simulink model "Truck_model_step"  (R2025a)
settings: Solver=VariableStepAuto  StartTime=0.0  StopTime=30  RelTol=1e-3
values from neighbouring files (symbols this model uses):
  A = [zeros(10) eye(10) ... (first row only)    [New_method_with_static_Equilibrium.m]    (also in PeakForce_and_Amp.m; Rough_work.m = [0 1 0 0 0 0 0 0 0 0 0 0 0 0 0 0 0 0 0 0; Rough_work_sweep.m = [0 1 0 0 0 0 0 0 0 0 0 0 0 0 0 0 0 0 0 0)
  B = [0 0 0 0 ... (first row only)    [New_method_with_static_Equilibrium.m]    (also in PeakForce_and_Amp.m; Rough_work.m; Rough_work_sweep.m)
  C = [-(Csf+Csr+Csd) Csf Csr (-Csr*lr+Csf*lf-Csd*a1) 0 0 0 0 Csd -Csd*lfd ... (first row only)    [New_method_with_static_Equilibrium.m]    (also in PeakForce_and_Amp.m; Rough_work.m = eye(20); Rough_work_sweep.m = eye(20))
  D = zeros(20,4)    [New_method_with_static_Equilibrium.m]    (also in PeakForce_and_Amp.m; Rough_work.m; Rough_work_sweep.m)
  t1 = s1/Vx    (= 0.06825)    [New_method_with_static_Equilibrium.m]    (also in PeakForce_and_Amp.m = s1/Vx; Rough_work.m = 0.1365; Rough_work_sweep.m = s1/Vx)
  t2 = s2/Vx    (= 0.34175)    [New_method_with_static_Equilibrium.m]    (also in PeakForce_and_Amp.m = s2/Vx; Rough_work.m = 0.6835; Rough_work_sweep.m = s2/Vx)
  t3 = s3/Vx    (= 0.66575)    [New_method_with_static_Equilibrium.m]    (also in PeakForce_and_Amp.m = s3/Vx; Rough_work.m = 1.3315; Rough_work_sweep.m = s3/Vx)
  t4 = s4/Vx    (= 1.01325)    [New_method_with_static_Equilibrium.m]    (also in PeakForce_and_Amp.m = s4/Vx; Rough_work.m = 2.0265; Rough_work_sweep.m = s4/Vx)
settings Model: Creator=lenovo  LastModifiedBy=lenovo

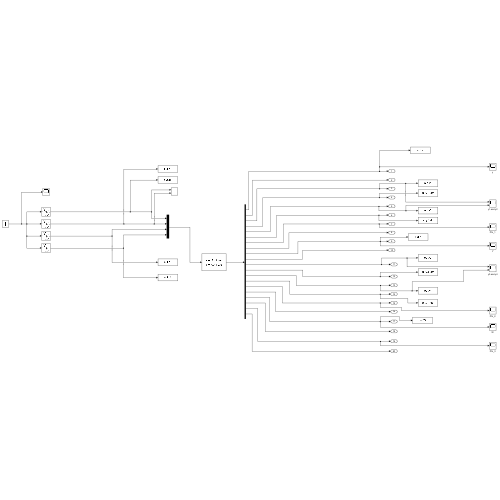
[thumbnail: Simulink's stored preview of the top-level diagram]
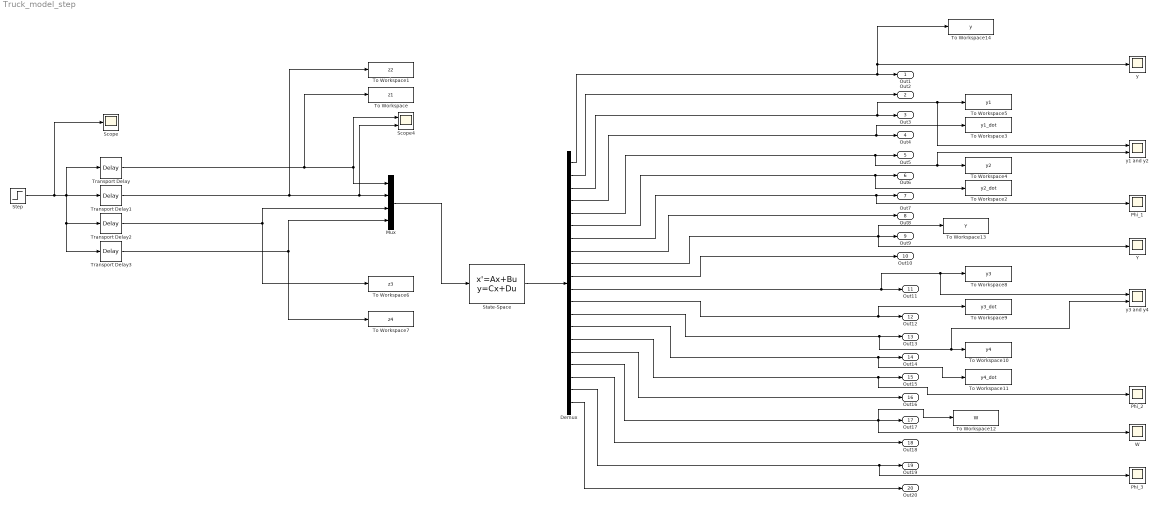
== system Truck_model_step ==
  Demux : Demux  Outputs=20
  Mux : Mux
  Phi_1 : Scope
      settings: ActiveDisplayYMinimum=-0.25192544075249879  ActiveDisplayYMaximum=0.21768735206441114  DataLoggingVariableName=ScopeData2
  Phi_2 : Scope
      settings: ActiveDisplayYMinimum=-0.0014235134101191549  ActiveDisplayYMaximum=0.0014402375247128129  DataLoggingVariableName=ScopeData9
  Phi_3 : Scope
      settings: ActiveDisplayYMinimum=-0.1066435087188474  ActiveDisplayYMaximum=0.11421754881493598  DataLoggingVariableName=ScopeData7
  Scope : Scope
      settings: ActiveDisplayYMinimum=-0.0020586486151432937  ActiveDisplayYMaximum=0.10161430322660607  DataLoggingVariableName=ScopeData8
  Scope4 : Scope  NumInputPorts=2
      settings: ActiveDisplayYMinimum=-1  ActiveDisplayYMaximum=1  DataLoggingVariableName=ScopeData4
  State-Space : StateSpace  A=A  B=B  C=C  D=D  InitialCondition=0
  Step : Step  After=0.03  SampleTime=0
  To Workspace : ToWorkspace  VariableName=z1  SaveFormat=Timeseries  SampleTime=-1
  To Workspace1 : ToWorkspace  VariableName=z2  SaveFormat=Timeseries  SampleTime=-1
  To Workspace10 : ToWorkspace  VariableName=y4  SaveFormat=Timeseries  SampleTime=-1
  To Workspace11 : ToWorkspace  VariableName=y4_dot  SaveFormat=Timeseries  SampleTime=-1
  To Workspace12 : ToWorkspace  VariableName=W  SaveFormat=Timeseries  SampleTime=-1
  To Workspace13 : ToWorkspace  VariableName=Y  SaveFormat=Timeseries  SampleTime=-1
  To Workspace14 : ToWorkspace  VariableName=y  SaveFormat=Timeseries  SampleTime=-1
  To Workspace2 : ToWorkspace  VariableName=y2_dot  SaveFormat=Timeseries  SampleTime=-1
  To Workspace3 : ToWorkspace  VariableName=y1_dot  SaveFormat=Timeseries  SampleTime=-1
  To Workspace4 : ToWorkspace  VariableName=y2  SaveFormat=Timeseries  SampleTime=-1
  To Workspace5 : ToWorkspace  VariableName=y1  SaveFormat=Timeseries  SampleTime=-1
  To Workspace6 : ToWorkspace  VariableName=z3  SaveFormat=Timeseries  SampleTime=-1
  To Workspace7 : ToWorkspace  VariableName=z4  SaveFormat=Timeseries  SampleTime=-1
  To Workspace8 : ToWorkspace  VariableName=y3  SaveFormat=Timeseries  SampleTime=-1
  To Workspace9 : ToWorkspace  VariableName=y3_dot  SaveFormat=Timeseries  SampleTime=-1
  Transport Delay : TransportDelay  DelayTime=t1  BufferSize=102400
  Transport Delay1 : TransportDelay  DelayTime=t2  BufferSize=102400
  Transport Delay2 : TransportDelay  DelayTime=t3  BufferSize=102400
  Transport Delay3 : TransportDelay  DelayTime=t4  BufferSize=102400
  W : Scope
      settings: ActiveDisplayYMinimum=-0.14455141261324181  ActiveDisplayYMaximum=0.15799358333233302  DataLoggingVariableName=ScopeData3
  Y : Scope
      settings: ActiveDisplayYMinimum=-0.17041377720557332  ActiveDisplayYMaximum=0.16739861220210034  DataLoggingVariableName=ScopeData5
  y : Scope
      settings: ActiveDisplayYMinimum=-0.061303830750307806  ActiveDisplayYMaximum=0.087715806737216392
  y1 and y2 : Scope  NumInputPorts=2
      settings: ActiveDisplayYMinimum=-0.01911712152421155  ActiveDisplayYMaximum=0.11666770112786763
  y3 and y4 : Scope  NumInputPorts=2
      settings: DataLoggingVariableName=ScopeData6
  Out1 : Outport
  Out2 : Outport  Port=2
  Out3 : Outport  Port=3
  Out4 : Outport  Port=4
  Out5 : Outport  Port=5
  Out6 : Outport  Port=6
  Out7 : Outport  Port=7
  Out8 : Outport  Port=8
  Out9 : Outport  Port=9
  Out10 : Outport  Port=10
  Out11 : Outport  Port=11
  Out12 : Outport  Port=12
  Out13 : Outport  Port=13
  Out14 : Outport  Port=14
  Out15 : Outport  Port=15
  Out16 : Outport  Port=16
  Out17 : Outport  Port=17
  Out18 : Outport  Port=18
  Out19 : Outport  Port=19
  Out20 : Outport  Port=20
  wires:
  Demux/1 -> y/1, To Workspace14/1, Out1/1
  Demux/11 -> y3 and y4/1, To Workspace8/1, Out11/1
  Demux/8 -> Out8/1
  Transport Delay/1 -> To Workspace/1, Scope4/1, Mux/1
  Demux/10 -> Out10/1
  Demux/20 -> Out20/1
  State-Space/1 -> Demux/1
  Mux/1 -> State-Space/1
  Demux/16 -> Out16/1
  Demux/14 -> To Workspace11/1, Out14/1
  Demux/17 -> To Workspace12/1, W/1, Out17/1
  Step/1 -> Transport Delay/1, Transport Delay1/1, Transport Delay3/1, Transport Delay2/1, Scope/1
  Demux/7 -> Phi_1/1, Out7/1
  Demux/9 -> To Workspace13/1, Y/1, Out9/1
  Demux/2 -> Out2/1
  Demux/5 -> To Workspace4/1, y1 and y2/2, Out5/1
  Demux/6 -> To Workspace2/1, Out6/1
  Demux/18 -> Out18/1
  Demux/3 -> y1 and y2/1, To Workspace5/1, Out3/1
  Demux/12 -> To Workspace9/1, Out12/1
  Transport Delay1/1 -> To Workspace1/1, Scope4/2, Mux/2
  Transport Delay2/1 -> Mux/3, To Workspace6/1
  Demux/4 -> To Workspace3/1, Out4/1
  Demux/13 -> y3 and y4/2, To Workspace10/1, Out13/1
  Demux/19 -> Phi_3/1, Out19/1
  Demux/15 -> Phi_2/1, Out15/1
  Transport Delay3/1 -> Mux/4, To Workspace7/1
